simulink model "exampleMSD"  (R2022b)
settings: Solver=FixedStepAuto  StartTime=0.0  StopTime=70  FixedStep=h  RelTol=1e-3
undefined symbols (not defined in the file): c, k, m, Ref_in
libraries: slpidlib x1
settings Model: Creator=Berkem Vural  LastModifiedBy=Claudia Yasar
settings DataIOCC: ReturnWorkspaceOutputs=off
settings OptimizationCC: ReuseModelBlockBuffer=on

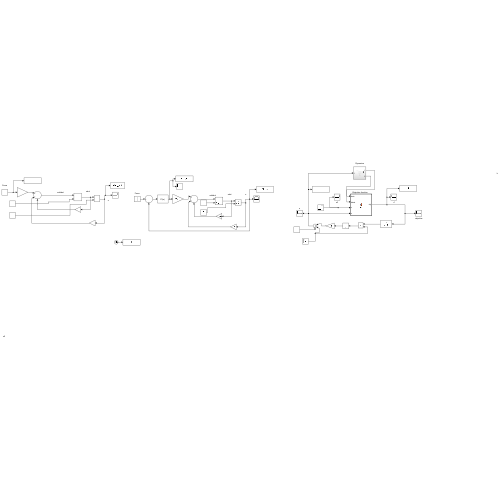
[thumbnail: Simulink's stored preview of the top-level diagram]
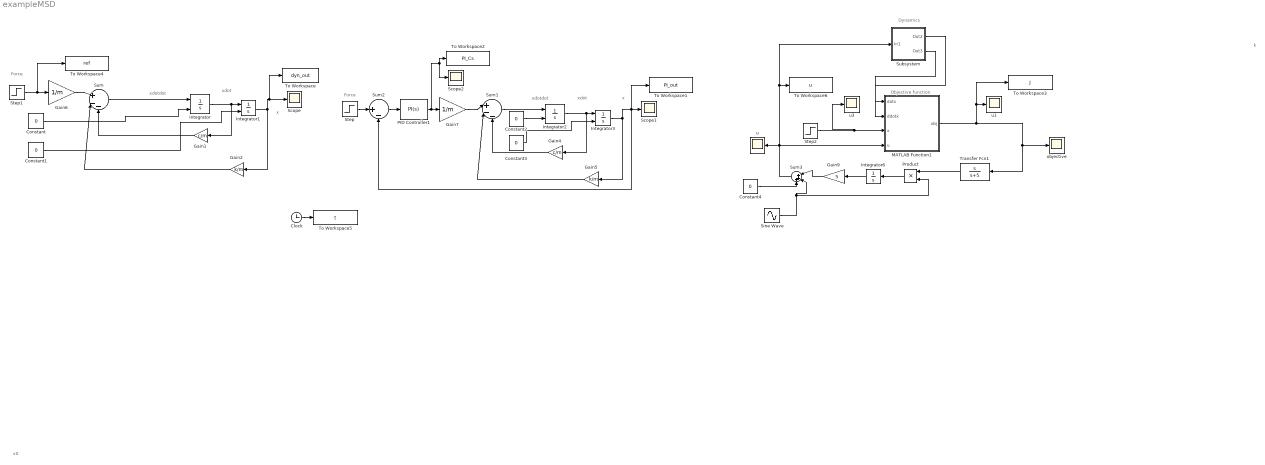
== system exampleMSD ==
  note: Objective function
  note: Dynamics
  note: Force
  note: k
  note: xdot
  note: xdotdot
  note: xdotdot
  note: xdot
  note: x0
  note: x
  note: x
  note: Force
  Clock : Clock
  Constant{,1..4} (5 alike) : Constant  Value=0
  Gain1 : Gain  Gain=c/m
  Gain2 : Gain  Gain=k/m
  Gain4 : Gain  Gain=c/m
  Gain5 : Gain  Gain=k/m
  Gain6 : Gain  Gain=1/m
  Gain7 : Gain  Gain=1/m
  Gain9 : Gain  Gain=5
  Integrator : Integrator  InitialConditionSource=external  InitialCondition=1
  Integrator1 : Integrator  InitialConditionSource=external
  Integrator2 : Integrator  InitialConditionSource=external  InitialCondition=1
  Integrator3 : Integrator  InitialConditionSource=external
  Integrator6 : Integrator
  MATLAB Function1 : MATLAB Function  TreatAsAtomicUnit=on
  PID Controller1 : slpidlib/PID Controller  Controller=PI  Form=Parallel  TimeDomain=Continuous-time  UseExternalTs=off  SampleTime=-1  IntegratorMethod=Forward Euler  FilterMethod=Forward Euler  ControllerParametersSource=internal  P=0.2  I=0.091236871879019  UseKiTs=off  D=0  N=100  UseFilter=on  TunerSelectOption=Transfer Function Based (PID Tuner App)  InitialConditionSource=internal  InitialConditionForIntegrator=0  InitialConditionForFilter=0  DifferentiatorICPrevScaledInput=0  ExternalReset=none  TrackingMode=off  Kt=1  LimitOutput=off  SatLimitsSource=internal  UpperSaturationLimit=inf  LowerSaturationLimit=-inf  LinearizeAsGain=on  AntiWindupMode=none  Kb=1  LimitIntegrator=off  UpperIntegratorSaturationLimit=inf  LowerIntegratorSaturationLimit=-inf  POutMin=[]  POutMax=[]  IOutMin=[]  IOutMax=[]  DOutMin=[]  DOutMax=[]  NOutMin=[]  NOutMax=[]  SumOutMin=[]  SumOutMax=[]  SaturationOutMin=[]  SaturationOutMax=[]  PParamMin=[]  PParamMax=[]  IParamMin=[]  IParamMax=[]  DParamMin=[]  DParamMax=[]  NParamMin=[]  NParamMax=[]  KbParamMin=[]  KbParamMax=[]  KtParamMin=[]  KtParamMax=[]  KbOutMin=[]  KbOutMax=[]  KtOutMin=[]  KtOutMax=[]  IntegratorOutMin=[]  IntegratorOutMax=[]  FilterOutMin=[]  FilterOutMax=[]  SumI1OutMin=[]  SumI1OutMax=[]  SumI2OutMin=[]  SumI2OutMax=[]  SumI3OutMin=[]  SumI3OutMax=[]  SumI4OutMin=[]  SumI4OutMax=[]  SumDOutMin=[]  SumDOutMax=[]  DifferentiatorOutMin=[]  DifferentiatorOutMax=[]  FilterDiffOutCoefMin=[]  FilterDiffOutCoefMax=[]  ReciprocalOutMin=[]  ReciprocalOutMax=[]  SumDenOutMin=[]  SumDenOutMax=[]  SumNumOutMin=[]  SumNumOutMax=[]  DivideOutMin=[]  DivideOutMax=[]  UdiffTsProdOutMin=[]  UdiffTsProdOutMax=[]  NTsProdOutMin=[]  NTsProdOutMax=[]  UintegralTsProdOutMin=[]  UintegralTsProdOutMax=[]  UngainTsProdOutMin=[]  UngainTsProdOutMax=[]  ClampingZeroOutDataTypeStr=Inherit: Inherit via back propagation  ClampingZeroOutMin=[]  ClampingZeroOutMax=[]  FilterDenConstantOutDataTypeStr=Inherit: Inherit via back propagation  FilterDenConstantOutMin=[]  FilterDenConstantOutMax=[]  PCopyOutDataTypeStr=Inherit: Inherit via back propagation  PCopyOutMin=[]  PCopyOutMax=[]  NCopyOutDataTypeStr=Inherit: Inherit via back propagation  NCopyOutMin=[]  NCopyOutMax=[]  IntegratorContinuousStateAttributes=''  IntegratorStateMustResolveToSignalObject=off  IntegratorRTWStateStorageClass=Auto  FilterContinuousStateAttributes=''  FilterStateMustResolveToSignalObject=off  FilterRTWStateStorageClass=Auto  ParallelPVariant=InternalParameters  IdealPVariant=Disabled  IVariant=InternalParameters  DVariant=Disabled  IntegratorVariant=Continuous  SatVariant=Disabled  AWVariant=Passthrough  PCopyVariant=Disabled  TRVariant=Disabled  FdbkBlocksVariant=Forward  IdealPFdbkVariant=Disabled  SatFdbkVariant=Disabled  DerivativeFilterVariant=Disabled  NVariant=Disabled  NCopyVariant=Disabled_SignalSpec  FilterICVariant=Disabled  IntegratorICVariant=InternalICs  ExternalResetVariant=Disabled  TRSumVariant=Passthrough  SumFdbkVariant=Disabled  SumVariant=Sum_PI  TsampFilterVariant=InternalTs  TsampNgainVariant=Passthrough  TsampIntegralVariant=Passthrough  ExternalSaturationOutDataTypeStr=Inherit: Same as second input
  Product : Product
  Scope : Scope
  Scope1 : Scope
  Scope2 : Scope
  Sine Wave : Sin  Amplitude=0.03  Frequency=8  SampleTime=0
  Step : Step  After=Ref_in  SampleTime=0
  Step1 : Step  After=Ref_in  SampleTime=0
  Step2 : Step  Time=0  After=Ref_in  SampleTime=0
  Subsystem : Subsystem
  Sum : Sum  Inputs=|+--
  Sum1 : Sum  Inputs=|+--
  Sum2 : Sum  Inputs=|+-
  Sum3 : Sum  Inputs=|+++
  To Workspace : ToWorkspace  VariableName=dyn_out  SampleTime=-1
  To Workspace1 : ToWorkspace  VariableName=PI_out  SampleTime=-1
      settings: Save2DSignal=2-D array (concatenate along first dimension)
  To Workspace2 : ToWorkspace  VariableName=PI_Cs  SampleTime=-1
      settings: Save2DSignal=2-D array (concatenate along first dimension)
  To Workspace3 : ToWorkspace  VariableName=J  SampleTime=-1
      settings: Save2DSignal=2-D array (concatenate along first dimension)
  To Workspace4 : ToWorkspace  VariableName=ref  SampleTime=-1
  To Workspace5 : ToWorkspace  VariableName=t  SampleTime=-1
  To Workspace6 : ToWorkspace  VariableName=u  SampleTime=-1
      settings: Save2DSignal=2-D array (concatenate along first dimension)
  Transfer Fcn1 : TransferFcn  Numerator=[1 0]  Denominator=[1 5]
  objective : Scope
  u : Scope
  u1 : Scope
  u3 : Scope
  wires:
  Sum/1 -> Integrator/1
  Integrator/1 -> Integrator1/1, Gain1/1
  Gain1/1 -> Sum/3
  Integrator1/1 -> To Workspace/1, Scope/1, Gain2/1
  Gain2/1 -> Sum/2
  Step1/1 -> To Workspace4/1, Gain6/1
  Constant/1 -> Integrator/2
  Constant1/1 -> Integrator1/2
  Constant2/1 -> Integrator2/2
  Constant3/1 -> Integrator3/2
  Sum1/1 -> Integrator2/1
  Gain5/1 -> Sum1/2
  Gain4/1 -> Sum1/3
  Integrator2/1 -> Integrator3/1, Gain4/1
  Product/1 -> Integrator6/1
  Integrator6/1 -> Gain9/1
  Gain9/1 -> Sum3/1
  Sine Wave/1 -> Product/2, Sum3/2
  Transfer Fcn1/1 -> Product/1
  MATLAB Function1/1(obj) -> To Workspace3/1, u1/1, objective/1, Transfer Fcn1/1
  Step/1 -> Sum2/1
  Sum2/1 -> PID Controller1/1
  Integrator3/1 -> Sum2/2, To Workspace1/1, Scope1/1, Gain5/1
  Gain6/1 -> Sum/1
  Gain7/1 -> Sum1/1
  PID Controller1/1 -> Scope2/1, To Workspace2/1, Gain7/1
  Step2/1 -> u3/1, MATLAB Function1/3(x)
  Subsystem/1(Out2) -> MATLAB Function1/1(dotx)
  Subsystem/2(Out3) -> MATLAB Function1/2(ddotx)
  Constant4/1 -> Sum3/3
  Sum3/1 -> To Workspace6/1, Subsystem/1(In1), u/1, MATLAB Function1/4(u)
  Clock/1 -> To Workspace5/1

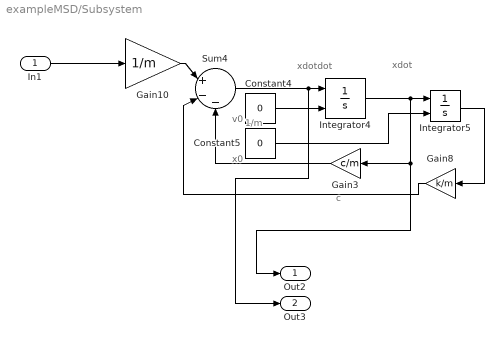
== system exampleMSD/Subsystem ==
  note: v0
  note: x0
  note: xdot
  note: c
  note: xdotdot
  note: 1/m
  In1 : Inport
  Constant4 : Constant  Value=0
  Constant5 : Constant  Value=0
  Gain10 : Gain  Gain=1/m
  Gain3 : Gain  Gain=c/m
  Gain8 : Gain  Gain=k/m
  Integrator4 : Integrator  InitialConditionSource=external  InitialCondition=1
  Integrator5 : Integrator  InitialConditionSource=external
  Sum4 : Sum  Inputs=|+--
  Out2 : Outport
  Out3 : Outport  Port=2
  wires:
  Integrator4/1 -> Integrator5/1, Out2/1, Gain3/1
  Constant4/1 -> Integrator4/2
  Gain10/1 -> Sum4/1
  Integrator5/1 -> Gain8/1
  Sum4/1 -> Out3/1, Integrator4/1
  Constant5/1 -> Integrator5/2
  Gain3/1 -> Sum4/3
  Gain8/1 -> Sum4/2
  In1/1 -> Gain10/1

== matlab function exampleMSD/MATLAB Function1 ==
  data: dotx input; ddotx input; x input; u input; obj output




function obj = fcn(dotx, ddotx,x,u)

 m=2;
 c=0.5;
 k=1;

obj=(x-(u-c*dotx-m*ddotx)/k);

end
